simulink model "simulink_Comparison_Plot"  (R2020a)
settings: Solver=ode4  StartTime=0.0  StopTime=10.0  FixedStep=0.01  RelTol=1e-3
settings Model: Creator=Juan Augusto Paredes  LastModifiedBy=Juan Augusto Paredes

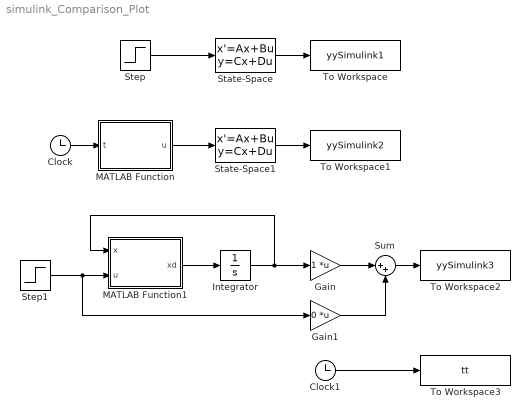
== system simulink_Comparison_Plot ==
  Clock : Clock
  Clock1 : Clock
  Gain : Gain  Multiplication=Matrix(K*u)
  Gain1 : Gain  Gain=0  Multiplication=Matrix(K*u)
  Integrator : Integrator  InitialCondition=2
  MATLAB Function : MATLAB Function  TreatAsAtomicUnit=on
  MATLAB Function1 : MATLAB Function  TreatAsAtomicUnit=on
  State-Space : StateSpace  A=-1  D=0  InitialCondition=2
  State-Space1 : StateSpace  A=-1  D=0  InitialCondition=2
  Step : Step  After=5  SampleTime=0
  Step1 : Step  After=5  SampleTime=0
  Sum : Sum  Inputs=|++
  To Workspace : ToWorkspace  VariableName=yySimulink1  SampleTime=-1
  To Workspace1 : ToWorkspace  VariableName=yySimulink2  SampleTime=-1
  To Workspace2 : ToWorkspace  VariableName=yySimulink3  SampleTime=-1
  To Workspace3 : ToWorkspace  VariableName=tt  SampleTime=-1
  wires:
  Gain1/1 -> Sum/2
  Clock/1 -> MATLAB Function/1(t)
  MATLAB Function1/1(xd) -> Integrator/1
  Integrator/1 -> Gain/1, MATLAB Function1/1(x)
  MATLAB Function/1(u) -> State-Space1/1
  Step/1 -> State-Space/1
  Step1/1 -> Gain1/1, MATLAB Function1/2(u)
  Gain/1 -> Sum/1
  State-Space/1 -> To Workspace/1
  State-Space1/1 -> To Workspace1/1
  Sum/1 -> To Workspace2/1
  Clock1/1 -> To Workspace3/1

== matlab function simulink_Comparison_Plot/MATLAB Function ==
  data: t input; u output
function u = stepFun(t)
    u = 5.*(t>=1);
end

== matlab function simulink_Comparison_Plot/MATLAB Function1 ==
  data: x input; u input; xd output
function xd = odefun(x, u)

    A = -1;
    B = 1;

    xd = A*x + B*u;

end
